simulink library "motion"  (Simulink 4.00)
undefined symbols (not defined in the file or in its folder): A6, Ac, Acd, ad, Aff, Aff0, Aff6, Ap, As, B6, Bc, Bcd, Bff, Bff0, Bff6, Bp, Bs, C6, Cc, Ccd, Cff, Cff0, Cff6, Cp, Cs, D6, Dc, dd, Ddd, Dff, Dff0, Dff6, Dp, Ds, jd, Ts, Tsettle
libraries: motion x5
(part 4 of 4)

== system motion/Real Time/Plan Trajectory (with displays)/Round up7 ==
  In1 : Inport  Port=1
  Product : Product  Inputs=*/  Multiplication=Element-wise(.*)  SaturateOnIntegerOverflow=on
  Product1 : Product  Inputs=**  Multiplication=Element-wise(.*)  SaturateOnIntegerOverflow=on
  Round up : Rounding  Operator=ceil
  Out1 : Outport  Port=1
  wires:
  [Ts] -> Product1/2, Product/2
  Product/1 -> Round up/1
  Round up/1 -> Product1/1
  In1/1 -> Product/1
  Product1/1 -> Out1/1

== system motion/Real Time/Plan Trajectory (with displays)/Round up8 ==
  In1 : Inport  Port=1
  Product : Product  Inputs=*/  Multiplication=Element-wise(.*)  SaturateOnIntegerOverflow=on
  Product1 : Product  Inputs=**  Multiplication=Element-wise(.*)  SaturateOnIntegerOverflow=on
  Round up : Rounding  Operator=ceil
  Out1 : Outport  Port=1
  wires:
  Product1/1 -> Out1/1
  In1/1 -> Product/1
  Round up/1 -> Product1/1
  Product/1 -> Round up/1
  [Ts] -> Product/2, Product1/2

== system motion/Real Time/Plan Trajectory (with displays)/Round up9 ==
  In1 : Inport  Port=1
  Product : Product  Inputs=*/  Multiplication=Element-wise(.*)  SaturateOnIntegerOverflow=on
  Product1 : Product  Inputs=**  Multiplication=Element-wise(.*)  SaturateOnIntegerOverflow=on
  Round up : Rounding  Operator=ceil
  Out1 : Outport  Port=1
  wires:
  [Ts] -> Product1/2, Product/2
  Product/1 -> Round up/1
  Round up/1 -> Product1/1
  In1/1 -> Product/1
  Product1/1 -> Out1/1

== system motion/Real Time/Plan Trajectory (with displays)/ta amax ==
  u : Inport  Port=1
  dd : Inport  Port=2
  Mux1 : Mux  Inputs=3
  Mux17 : Mux  Inputs=3
  c1 : Fcn  Expr=u(1)*(u(1)+u(2))
  c2 : Fcn  Expr=3*u(1)*( 2*u(1)^2 + u(2)*(3*u(1) + u(2)) )
  c3 : Fcn  Expr=2*u(1)*( u(1)*( 4*u(1)^2 + u(2)*(8*u(1) + 5*u(2)) ) + u(2)^3 )
  ta calc : Fcn  Expr=(-u(10) + sqrt(u(10)^2-4*u(9)*(u(11)-u(1)/u(8))))/(2*u(9))
  ta : Outport  Port=1
  c : Outport  Port=2
  wires:
  [dd] -> Mux1/2
  Mux17/1 -> c/1, [c]
  c1/1 -> Mux17/1
  c3/1 -> Mux17/3
  c2/1 -> Mux17/2
  ta calc/1 -> ta/1
  [c] -> Mux1/3
  [u] -> Mux1/1
  Mux1/1 -> ta calc/1
  [dd] -> c3/1, c2/1, c1/1
  dd/1 -> [dd]
  u/1 -> [u]

== system motion/Real Time/Plan Trajectory (with displays)/tj jmax ==
  u : Inport  Port=1
  dd : Inport  Port=2
  D : Fcn  Expr=sqrt(u(1)^3+u(2)^2)
  Demux : Demux  Outputs=5  BusSelectionMode=off
  Demux1 : Demux  Outputs=2  BusSelectionMode=off
  Mux1 : Mux  Inputs=2
  Mux12 : Mux  Inputs=2
  Mux2 : Mux  Inputs=2
  Mux3 : Mux  Inputs=3
  P : Fcn  Expr=-1/9*u(1)^2
  Q : Fcn  Expr=-1/27*u(1)^3-u(3)/(4*u(2)*u(1))
  R : Fcn  Expr=(-u(1)+u(2))^(1/3)
  Terminator{,1..4} (5 alike) : Terminator
  tj calc : Fcn  Expr=u(2) - u(1)/u(2) - 5/3*u(3)
  tj : Outport  Port=1
  wires:
  [td] -> Mux3/3
  tj calc/1 -> tj/1
  [R] -> Mux3/2
  [P] -> Mux3/1
  Mux3/1 -> tj calc/1
  R/1 -> [R]
  [D] -> Mux2/2
  [Q] -> Mux2/1
  Mux2/1 -> R/1
  D/1 -> [D]
  [Q] -> Mux1/2
  [P] -> Mux1/1
  Mux1/1 -> D/1
  Q/1 -> [Q]
  P/1 -> [P]
  [p] -> Mux12/2
  Mux12/1 -> Q/1
  [dd] -> Mux12/1, P/1
  Demux1/1 -> [td]
  Demux1/2 -> Terminator4/1  "dd"
  dd/1 -> [dd], Demux1/1
  Demux/5 -> Terminator3/1  "d"
  Demux/4 -> Terminator/1  "j"
  Demux/3 -> Terminator1/1  "a"
  Demux/2 -> Terminator2/1  "v"
  Demux/1 -> [p]
  u/1 -> Demux/1

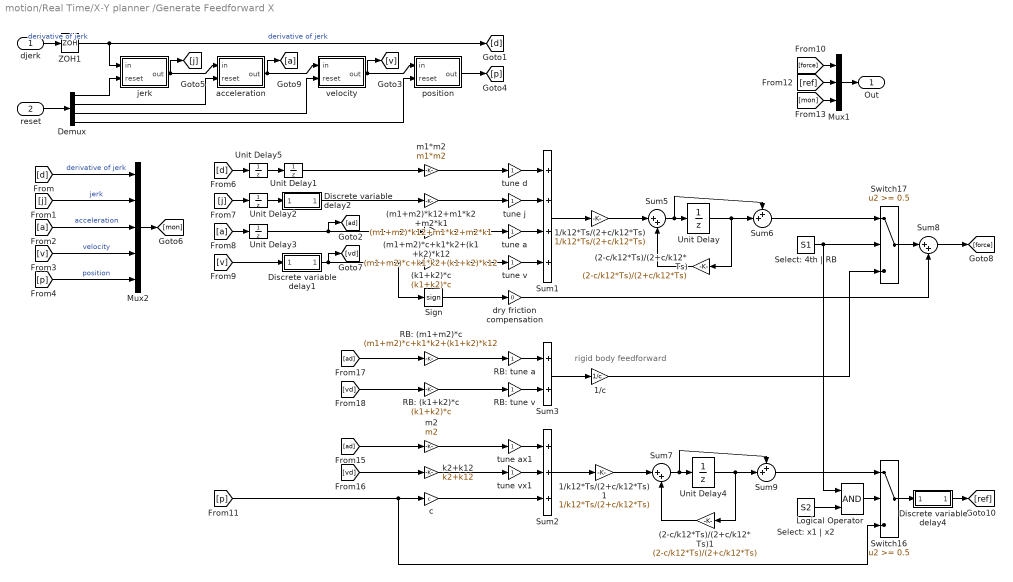
== system motion/Real Time/X-Y planner /Generate Feedforward X ==
  note: rigid body feedforward
  djerk : Inport  Port=1
  reset : Inport  Port=2
  (2-c/k12*Ts)/(2+c/k12*Ts) : Gain  Orientation=left  Gain=(2-c/k12*Ts)/(2+c/k12*Ts)  Multiplication=Element-wise(K.*u)  SaturateOnIntegerOverflow=on
  (2-c/k12*Ts)/(2+c/k12*Ts)1 : Gain  Orientation=left  Gain=(2-c/k12*Ts)/(2+c/k12*Ts)  Multiplication=Element-wise(K.*u)  SaturateOnIntegerOverflow=on
  (k1+k2)*c : Gain  Gain=(k1+k2)*c  Multiplication=Element-wise(K.*u)  SaturateOnIntegerOverflow=on
  (m1+m2)*c+k1*k2+(k1+k2)*k12 : Gain  Gain=(m1+m2)*c+k1*k2+(k1+k2)*k12  Multiplication=Element-wise(K.*u)  SaturateOnIntegerOverflow=on
  (m1+m2)*k12+m1*k2+m2*k1 : Gain  Gain=(m1+m2)*k12+m1*k2+m2*k1  Multiplication=Element-wise(K.*u)  SaturateOnIntegerOverflow=on
  1/c : Gain  Gain=1/c  Multiplication=Element-wise(K.*u)  SaturateOnIntegerOverflow=on
  1/k12*Ts/(2+c/k12*Ts) : Gain  Gain=1/k12*Ts/(2+c/k12*Ts)  Multiplication=Element-wise(K.*u)  SaturateOnIntegerOverflow=on
  1/k12*Ts/(2+c/k12*Ts)1 : Gain  Gain=1/k12*Ts/(2+c/k12*Ts)  Multiplication=Element-wise(K.*u)  SaturateOnIntegerOverflow=on
  Demux : Demux  Outputs=4  BusSelectionMode=off
  Discrete variable delay1 : Subsystem  mask{Ts=Ts, alpha=.5}
      mask prompts: Ts "Sample time"; alpha "Delay factor (between 0 and 1)"
      settings: RTWFcnNameOpts=Auto  RTWFileNameOpts=Auto
      mask Display: disp(sprintf('%3.1f*Ts',alpha))
  Discrete variable delay2 : Subsystem  mask{Ts=Ts, alpha=.5}
      mask prompts: Ts "Sample time"; alpha "Delay factor (between 0 and 1)"
      settings: RTWFcnNameOpts=Auto  RTWFileNameOpts=Auto
      mask Display: disp(sprintf('%3.1f*Ts',alpha))
  Discrete variable delay4 : Subsystem  mask{Ts=Ts, alpha=.5}
      mask prompts: Ts "Sample time"; alpha "Delay factor (between 0 and 1)"
      settings: RTWFcnNameOpts=Auto  RTWFileNameOpts=Auto
      mask Display: disp(sprintf('%3.1f*Ts',alpha))
  Logical Operator : Logic  Operator=AND  Inputs=2
  Mux1 : Mux  Inputs=3
  Mux2 : Mux  Inputs=5
  RB: (k1+k2)*c : Gain  Gain=(k1+k2)*c  Multiplication=Element-wise(K.*u)  SaturateOnIntegerOverflow=on
  RB: (m1+m2)*c : Gain  Gain=(m1+m2)*c+k1*k2+(k1+k2)*k12  Multiplication=Element-wise(K.*u)  SaturateOnIntegerOverflow=on
  RB: tune a : Gain  Gain=1  Multiplication=Element-wise(K.*u)  SaturateOnIntegerOverflow=on
  RB: tune v : Gain  Gain=1  Multiplication=Element-wise(K.*u)  SaturateOnIntegerOverflow=on
  Select: 4th | RB : Constant  Value=S1
  Select: x1 | x2 : Constant  Value=S2
  Sign : Signum
  Sum1 : Sum  Inputs=++++  SaturateOnIntegerOverflow=on
  Sum2 : Sum  Inputs=+++  SaturateOnIntegerOverflow=on
  Sum3 : Sum  Inputs=++  SaturateOnIntegerOverflow=on
  Sum5 : Sum  Inputs=|++  SaturateOnIntegerOverflow=on
  Sum6 : Sum  Inputs=++|  SaturateOnIntegerOverflow=on
  Sum7 : Sum  Inputs=|++  SaturateOnIntegerOverflow=on
  Sum8 : Sum  Inputs=|++  SaturateOnIntegerOverflow=on
  Sum9 : Sum  Inputs=++|  SaturateOnIntegerOverflow=on
  Switch16 : Switch  Threshold=0.5
  Switch17 : Switch  Threshold=0.5
  Unit Delay{,1..5} (6 alike) : UnitDelay  X0=0  SampleTime=Ts
  ZOH1 : ZeroOrderHold  SampleTime=Ts
  acceleration : Subsystem
      settings: RTWFcnNameOpts=Auto  RTWFileNameOpts=Auto
  c : Gain  Gain=c  Multiplication=Element-wise(K.*u)  SaturateOnIntegerOverflow=on
  dry friction compensation : Gain  Gain=0  Multiplication=Element-wise(K.*u)  SaturateOnIntegerOverflow=on
  jerk : Subsystem
      settings: RTWFcnNameOpts=Auto  RTWFileNameOpts=Auto
  k2+k12 : Gain  Gain=k2+k12  Multiplication=Element-wise(K.*u)  SaturateOnIntegerOverflow=on
  m1*m2 : Gain  Gain=m1*m2  Multiplication=Element-wise(K.*u)  SaturateOnIntegerOverflow=on
  m2 : Gain  Gain=m2  Multiplication=Element-wise(K.*u)  SaturateOnIntegerOverflow=on
  position : Subsystem
      settings: RTWFcnNameOpts=Auto  RTWFileNameOpts=Auto
  tune a : Gain  Gain=1  Multiplication=Element-wise(K.*u)  SaturateOnIntegerOverflow=on
  tune ax1 : Gain  Gain=1  Multiplication=Element-wise(K.*u)  SaturateOnIntegerOverflow=on
  tune d : Gain  Gain=1  Multiplication=Element-wise(K.*u)  SaturateOnIntegerOverflow=on
  tune j : Gain  Gain=1  Multiplication=Element-wise(K.*u)  SaturateOnIntegerOverflow=on
  tune v : Gain  Gain=1  Multiplication=Element-wise(K.*u)  SaturateOnIntegerOverflow=on
  tune vx1 : Gain  Gain=1  Multiplication=Element-wise(K.*u)  SaturateOnIntegerOverflow=on
  velocity : Subsystem
      settings: RTWFcnNameOpts=Auto  RTWFileNameOpts=Auto
  Out : Outport  Port=1
  wires:
  c/1 -> Sum2/3
  Select: 4th | RB/1 -> Logical Operator/1, Switch17/2
  Sum9/1 -> Switch16/1
  1/c/1 -> Switch17/3
  dry friction compensation/1 -> Sum8/2
  Logical Operator/1 -> Switch16/2
  Select: x1 | x2/1 -> Logical Operator/2
  Discrete variable delay4/1(Out1) -> [ref]
  Switch16/1 -> Discrete variable delay4/1(In1)
  Sum8/1 -> [force]
  Switch17/1 -> Sum8/1
  Sum6/1 -> Switch17/1
  Unit Delay4/1 -> Sum9/2, (2-c/k12*Ts)/(2+c/k12*Ts)1/1
  Sum7/1 -> Sum9/1, Unit Delay4/1
  1/k12*Ts/(2+c/k12*Ts)1/1 -> Sum7/1
  Sum2/1 -> 1/k12*Ts/(2+c/k12*Ts)1/1
  (2-c/k12*Ts)/(2+c/k12*Ts)1/1 -> Sum7/2
  [vd] -> k2+k12/1
  [ad] -> m2/1
  [p] -> c/1, Switch16/3
  m2/1 -> tune ax1/1
  tune ax1/1 -> Sum2/1
  k2+k12/1 -> tune vx1/1
  tune vx1/1 -> Sum2/2
  [ad] -> RB: (m1+m2)*c/1
  [vd] -> RB: (k1+k2)*c/1
  RB: (m1+m2)*c/1 -> RB: tune a/1
  RB: tune a/1 -> Sum3/1
  RB: (k1+k2)*c/1 -> RB: tune v/1
  RB: tune v/1 -> Sum3/2
  Sum3/1 -> 1/c/1
  [force] -> Mux1/1
  [ref] -> Mux1/2
  [mon] -> Mux1/3
  Mux1/1 -> Out/1
  Unit Delay3/1 -> [ad], (m1+m2)*c+k1*k2+(k1+k2)*k12/1
  Discrete variable delay2/1(Out1) -> (m1+m2)*k12+m1*k2+m2*k1/1
  Unit Delay1/1 -> m1*m2/1
  m1*m2/1 -> tune d/1
  tune d/1 -> Sum1/1
  (m1+m2)*k12+m1*k2+m2*k1/1 -> tune j/1
  tune j/1 -> Sum1/2
  (m1+m2)*c+k1*k2+(k1+k2)*k12/1 -> tune a/1
  tune a/1 -> Sum1/3
  (k1+k2)*c/1 -> tune v/1
  tune v/1 -> Sum1/4
  Unit Delay/1 -> Sum6/2, (2-c/k12*Ts)/(2+c/k12*Ts)/1
  Sum5/1 -> Sum6/1, Unit Delay/1
  1/k12*Ts/(2+c/k12*Ts)/1 -> Sum5/1
  Sum1/1 -> 1/k12*Ts/(2+c/k12*Ts)/1
  (2-c/k12*Ts)/(2+c/k12*Ts)/1 -> Sum5/2
  Sign/1 -> dry friction compensation/1
  djerk/1 -> ZOH1/1  "derivative of jerk"
  Unit Delay2/1 -> Discrete variable delay2/1(In1)
  Unit Delay5/1 -> Unit Delay1/1
  [v] -> Discrete variable delay1/1(In1)
  [a] -> Unit Delay3/1
  [j] -> Unit Delay2/1
  [d] -> Unit Delay5/1
  [v] -> Mux2/4  "velocity"
  [a] -> Mux2/3  "acceleration"
  [j] -> Mux2/2  "jerk"
  [d] -> Mux2/1  "derivative of jerk"
  [p] -> Mux2/5  "position"
  Mux2/1 -> [mon]
  reset/1 -> Demux/1
  ZOH1/1 -> jerk/1(in), [d]  "derivative of jerk"
  acceleration/1(out) -> [a], velocity/1(in)
  jerk/1(out) -> [j], acceleration/1(in)
  Demux/1 -> jerk/2(reset)
  Demux/2 -> acceleration/2(reset)
  Demux/3 -> velocity/2(reset)
  velocity/1(out) -> [v], position/1(in)
  Demux/4 -> position/2(reset)
  Discrete variable delay1/1(Out1) -> [vd], (k1+k2)*c/1, Sign/1
  position/1(out) -> [p]

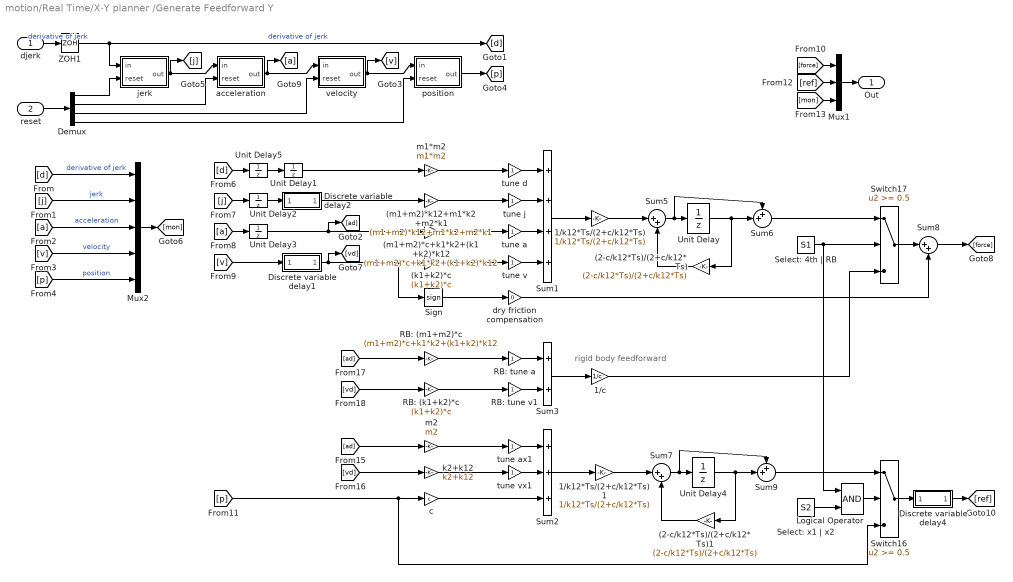
== system motion/Real Time/X-Y planner /Generate Feedforward Y ==
  note: rigid body feedforward
  djerk : Inport  Port=1
  reset : Inport  Port=2
  (2-c/k12*Ts)/(2+c/k12*Ts) : Gain  Orientation=left  Gain=(2-c/k12*Ts)/(2+c/k12*Ts)  Multiplication=Element-wise(K.*u)  SaturateOnIntegerOverflow=on
  (2-c/k12*Ts)/(2+c/k12*Ts)1 : Gain  Orientation=left  Gain=(2-c/k12*Ts)/(2+c/k12*Ts)  Multiplication=Element-wise(K.*u)  SaturateOnIntegerOverflow=on
  (k1+k2)*c : Gain  Gain=(k1+k2)*c  Multiplication=Element-wise(K.*u)  SaturateOnIntegerOverflow=on
  (m1+m2)*c+k1*k2+(k1+k2)*k12 : Gain  Gain=(m1+m2)*c+k1*k2+(k1+k2)*k12  Multiplication=Element-wise(K.*u)  SaturateOnIntegerOverflow=on
  (m1+m2)*k12+m1*k2+m2*k1 : Gain  Gain=(m1+m2)*k12+m1*k2+m2*k1  Multiplication=Element-wise(K.*u)  SaturateOnIntegerOverflow=on
  1/c : Gain  Gain=1/c  Multiplication=Element-wise(K.*u)  SaturateOnIntegerOverflow=on
  1/k12*Ts/(2+c/k12*Ts) : Gain  Gain=1/k12*Ts/(2+c/k12*Ts)  Multiplication=Element-wise(K.*u)  SaturateOnIntegerOverflow=on
  1/k12*Ts/(2+c/k12*Ts)1 : Gain  Gain=1/k12*Ts/(2+c/k12*Ts)  Multiplication=Element-wise(K.*u)  SaturateOnIntegerOverflow=on
  Demux : Demux  Outputs=4  BusSelectionMode=off
  Discrete variable delay1 : Subsystem  mask{Ts=Ts, alpha=.5}
      mask prompts: Ts "Sample time"; alpha "Delay factor (between 0 and 1)"
      settings: RTWFcnNameOpts=Auto  RTWFileNameOpts=Auto
      mask Display: disp(sprintf('%3.1f*Ts',alpha))
  Discrete variable delay2 : Subsystem  mask{Ts=Ts, alpha=.5}
      mask prompts: Ts "Sample time"; alpha "Delay factor (between 0 and 1)"
      settings: RTWFcnNameOpts=Auto  RTWFileNameOpts=Auto
      mask Display: disp(sprintf('%3.1f*Ts',alpha))
  Discrete variable delay4 : Subsystem  mask{Ts=Ts, alpha=.5}
      mask prompts: Ts "Sample time"; alpha "Delay factor (between 0 and 1)"
      settings: RTWFcnNameOpts=Auto  RTWFileNameOpts=Auto
      mask Display: disp(sprintf('%3.1f*Ts',alpha))
  Logical Operator : Logic  Operator=AND  Inputs=2
  Mux1 : Mux  Inputs=3
  Mux2 : Mux  Inputs=5
  RB: (k1+k2)*c : Gain  Gain=(k1+k2)*c  Multiplication=Element-wise(K.*u)  SaturateOnIntegerOverflow=on
  RB: (m1+m2)*c : Gain  Gain=(m1+m2)*c+k1*k2+(k1+k2)*k12  Multiplication=Element-wise(K.*u)  SaturateOnIntegerOverflow=on
  RB: tune a : Gain  Gain=1  Multiplication=Element-wise(K.*u)  SaturateOnIntegerOverflow=on
  RB: tune v1 : Gain  Gain=1  Multiplication=Element-wise(K.*u)  SaturateOnIntegerOverflow=on
  Select: 4th | RB : Constant  Value=S1
  Select: x1 | x2 : Constant  Value=S2
  Sign : Signum
  Sum1 : Sum  Inputs=++++  SaturateOnIntegerOverflow=on
  Sum2 : Sum  Inputs=+++  SaturateOnIntegerOverflow=on
  Sum3 : Sum  Inputs=++  SaturateOnIntegerOverflow=on
  Sum5 : Sum  Inputs=|++  SaturateOnIntegerOverflow=on
  Sum6 : Sum  Inputs=++|  SaturateOnIntegerOverflow=on
  Sum7 : Sum  Inputs=|++  SaturateOnIntegerOverflow=on
  Sum8 : Sum  Inputs=|++  SaturateOnIntegerOverflow=on
  Sum9 : Sum  Inputs=++|  SaturateOnIntegerOverflow=on
  Switch16 : Switch  Threshold=0.5
  Switch17 : Switch  Threshold=0.5
  Unit Delay{,1..5} (6 alike) : UnitDelay  X0=0  SampleTime=Ts
  ZOH1 : ZeroOrderHold  SampleTime=Ts
  acceleration : Subsystem
      settings: RTWFcnNameOpts=Auto  RTWFileNameOpts=Auto
  c : Gain  Gain=c  Multiplication=Element-wise(K.*u)  SaturateOnIntegerOverflow=on
  dry friction compensation : Gain  Gain=0  Multiplication=Element-wise(K.*u)  SaturateOnIntegerOverflow=on
  jerk : Subsystem
      settings: RTWFcnNameOpts=Auto  RTWFileNameOpts=Auto
  k2+k12 : Gain  Gain=k2+k12  Multiplication=Element-wise(K.*u)  SaturateOnIntegerOverflow=on
  m1*m2 : Gain  Gain=m1*m2  Multiplication=Element-wise(K.*u)  SaturateOnIntegerOverflow=on
  m2 : Gain  Gain=m2  Multiplication=Element-wise(K.*u)  SaturateOnIntegerOverflow=on
  position : Subsystem
      settings: RTWFcnNameOpts=Auto  RTWFileNameOpts=Auto
  tune a : Gain  Gain=1  Multiplication=Element-wise(K.*u)  SaturateOnIntegerOverflow=on
  tune ax1 : Gain  Gain=1  Multiplication=Element-wise(K.*u)  SaturateOnIntegerOverflow=on
  tune d : Gain  Gain=1  Multiplication=Element-wise(K.*u)  SaturateOnIntegerOverflow=on
  tune j : Gain  Gain=1  Multiplication=Element-wise(K.*u)  SaturateOnIntegerOverflow=on
  tune v : Gain  Gain=1  Multiplication=Element-wise(K.*u)  SaturateOnIntegerOverflow=on
  tune vx1 : Gain  Gain=1  Multiplication=Element-wise(K.*u)  SaturateOnIntegerOverflow=on
  velocity : Subsystem
      settings: RTWFcnNameOpts=Auto  RTWFileNameOpts=Auto
  Out : Outport  Port=1
  wires:
  position/1(out) -> [p]
  Discrete variable delay1/1(Out1) -> Sign/1, (k1+k2)*c/1, [vd]
  Demux/4 -> position/2(reset)
  velocity/1(out) -> position/1(in), [v]
  Demux/3 -> velocity/2(reset)
  Demux/2 -> acceleration/2(reset)
  Demux/1 -> jerk/2(reset)
  jerk/1(out) -> acceleration/1(in), [j]
  acceleration/1(out) -> velocity/1(in), [a]
  ZOH1/1 -> [d], jerk/1(in)  "derivative of jerk"
  reset/1 -> Demux/1
  Mux2/1 -> [mon]
  [p] -> Mux2/5  "position"
  [d] -> Mux2/1  "derivative of jerk"
  [j] -> Mux2/2  "jerk"
  [a] -> Mux2/3  "acceleration"
  [v] -> Mux2/4  "velocity"
  [d] -> Unit Delay5/1
  [j] -> Unit Delay2/1
  [a] -> Unit Delay3/1
  [v] -> Discrete variable delay1/1(In1)
  Unit Delay5/1 -> Unit Delay1/1
  Unit Delay2/1 -> Discrete variable delay2/1(In1)
  djerk/1 -> ZOH1/1  "derivative of jerk"
  Sign/1 -> dry friction compensation/1
  (2-c/k12*Ts)/(2+c/k12*Ts)/1 -> Sum5/2
  Sum1/1 -> 1/k12*Ts/(2+c/k12*Ts)/1
  1/k12*Ts/(2+c/k12*Ts)/1 -> Sum5/1
  Sum5/1 -> Unit Delay/1, Sum6/1
  Unit Delay/1 -> (2-c/k12*Ts)/(2+c/k12*Ts)/1, Sum6/2
  tune v/1 -> Sum1/4
  (k1+k2)*c/1 -> tune v/1
  tune a/1 -> Sum1/3
  (m1+m2)*c+k1*k2+(k1+k2)*k12/1 -> tune a/1
  tune j/1 -> Sum1/2
  (m1+m2)*k12+m1*k2+m2*k1/1 -> tune j/1
  tune d/1 -> Sum1/1
  m1*m2/1 -> tune d/1
  Unit Delay1/1 -> m1*m2/1
  Discrete variable delay2/1(Out1) -> (m1+m2)*k12+m1*k2+m2*k1/1
  Unit Delay3/1 -> (m1+m2)*c+k1*k2+(k1+k2)*k12/1, [ad]
  Mux1/1 -> Out/1
  [mon] -> Mux1/3
  [ref] -> Mux1/2
  [force] -> Mux1/1
  Sum3/1 -> 1/c/1
  RB: tune v1/1 -> Sum3/2
  RB: (k1+k2)*c/1 -> RB: tune v1/1
  RB: tune a/1 -> Sum3/1
  RB: (m1+m2)*c/1 -> RB: tune a/1
  [vd] -> RB: (k1+k2)*c/1
  [ad] -> RB: (m1+m2)*c/1
  tune vx1/1 -> Sum2/2
  k2+k12/1 -> tune vx1/1
  tune ax1/1 -> Sum2/1
  m2/1 -> tune ax1/1
  [p] -> Switch16/3, c/1
  [ad] -> m2/1
  [vd] -> k2+k12/1
  (2-c/k12*Ts)/(2+c/k12*Ts)1/1 -> Sum7/2
  Sum2/1 -> 1/k12*Ts/(2+c/k12*Ts)1/1
  1/k12*Ts/(2+c/k12*Ts)1/1 -> Sum7/1
  Sum7/1 -> Unit Delay4/1, Sum9/1
  Unit Delay4/1 -> (2-c/k12*Ts)/(2+c/k12*Ts)1/1, Sum9/2
  Sum6/1 -> Switch17/1
  Switch17/1 -> Sum8/1
  Sum8/1 -> [force]
  Switch16/1 -> Discrete variable delay4/1(In1)
  Discrete variable delay4/1(Out1) -> [ref]
  Select: x1 | x2/1 -> Logical Operator/2
  Logical Operator/1 -> Switch16/2
  dry friction compensation/1 -> Sum8/2
  1/c/1 -> Switch17/3
  Sum9/1 -> Switch16/1
  Select: 4th | RB/1 -> Switch17/2, Logical Operator/1
  c/1 -> Sum2/3

== system motion/Real Time/X-Y planner /Waypoints ==
  start position : Inport  Port=1
  Trigger : TriggerPort  TriggerType=rising  OutputDataType=auto
  0 : Memory  X0=0  InheritSampleTime=on
  Constant1 : Constant  Value=pmin
  Constant2 : Constant  Value=1
  Constant3 : Constant  Value=0
  Constant4 : Constant  Value=0
  Memory : Memory  X0=0  InheritSampleTime=on
  Mux1 : Mux  Inputs=2
  Relational Operator : RelationalOperator  Operator=>
  Sum3 : Sum  Inputs=|+-  SaturateOnIntegerOverflow=on
  Switch{1..4} (4 alike) : Switch  Threshold=0.5
  distance : Fcn  Expr=sqrt( u(1)^2 + u(2)^2 )
  factor X : Fcn  Expr=u(2)/u(1)
  factor Y : Fcn  Expr=u(3)/u(1)
  positions : FromWorkspace  VariableName=X  SampleTime=-1  Interpolate=off  OutputAfterFinalValue=CyclicRepetition
  p : Outport  Port=1
  X : Outport  Port=2
  Y : Outport  Port=3
  pos : Outport  Port=4
  wires:
  Constant1/1 -> Switch4/1, Relational Operator/1
  Switch3/1 -> Y/1
  Switch2/1 -> X/1
  Switch4/1 -> p/1
  Relational Operator/1 -> Switch4/2, Switch3/2, Switch2/2
  Constant4/1 -> Switch3/1
  Constant3/1 -> Switch2/1
  factor Y/1 -> Switch3/3
  factor X/1 -> Switch2/3
  Switch1/1 -> Sum3/2
  Sum3/1 -> Mux1/2, distance/1
  Memory/1 -> Switch1/1
  start position/1 -> Switch1/3
  positions/1 -> pos/1, Memory/1, Sum3/1
  Mux1/1 -> factor Y/1, factor X/1
  distance/1 -> Switch4/3, Relational Operator/2, Mux1/1
  Constant2/1 -> 0/1
  0/1 -> Switch1/2

== system motion/Real Time/X-Y planner /single move  ==
  trigger : Inport  Port=1
  start : Inport  Port=2
  0 : Constant  Value=0
  0/1 : Saturate  UpperLimit=1  LowerLimit=0  LinearizeAsGain=on
  Logical Operator3 : Logic  Operator=OR  Inputs=2
  Memory1 : Memory  X0=0  InheritSampleTime=on
  Memory2 : Memory  X0=0  InheritSampleTime=on
  Sum : Sum  Inputs=|+-  SaturateOnIntegerOverflow=on
  Switch1 : Switch  Threshold=.5
  enable : Outport  Port=1
  wires:
  0/1 -> Switch1/1
  Switch1/1 -> Memory2/1
  start/1 -> Switch1/2
  0/1/1 -> Logical Operator3/1
  Logical Operator3/1 -> Switch1/3
  Memory2/1 -> Logical Operator3/2, enable/1
  trigger/1 -> Memory1/1, Sum/1
  Memory1/1 -> Sum/2
  Sum/1 -> 0/1/1

== system motion/Real Time/X-Y planner /Generate Feedforward X/Discrete variable delay1 ==
  In1 : Inport  Port=1
  1-alpha : Gain  Gain=1-alpha  Multiplication=Element-wise(K.*u)  SaturateOnIntegerOverflow=on
  Sum1 : Sum  Inputs=++|  SaturateOnIntegerOverflow=on
  Sum2 : Sum  Inputs=+-|  SaturateOnIntegerOverflow=on
  Unit Delay : UnitDelay  X0=0  SampleTime=Ts
  Out1 : Outport  Port=1
  wires:
  In1/1 -> Sum2/1, Unit Delay/1
  Unit Delay/1 -> Sum1/2, Sum2/2
  Sum1/1 -> Out1/1
  1-alpha/1 -> Sum1/1
  Sum2/1 -> 1-alpha/1

== system motion/Real Time/X-Y planner /Generate Feedforward X/Discrete variable delay2 ==
  In1 : Inport  Port=1
  1-alpha : Gain  Gain=1-alpha  Multiplication=Element-wise(K.*u)  SaturateOnIntegerOverflow=on
  Sum1 : Sum  Inputs=++|  SaturateOnIntegerOverflow=on
  Sum2 : Sum  Inputs=+-|  SaturateOnIntegerOverflow=on
  Unit Delay : UnitDelay  X0=0  SampleTime=Ts
  Out1 : Outport  Port=1
  wires:
  Sum2/1 -> 1-alpha/1
  1-alpha/1 -> Sum1/1
  Sum1/1 -> Out1/1
  Unit Delay/1 -> Sum2/2, Sum1/2
  In1/1 -> Unit Delay/1, Sum2/1

== system motion/Real Time/X-Y planner /Generate Feedforward X/Discrete variable delay4 ==
  In1 : Inport  Port=1
  1-alpha : Gain  Gain=1-alpha  Multiplication=Element-wise(K.*u)  SaturateOnIntegerOverflow=on
  Sum1 : Sum  Inputs=++|  SaturateOnIntegerOverflow=on
  Sum2 : Sum  Inputs=+-|  SaturateOnIntegerOverflow=on
  Unit Delay : UnitDelay  X0=0  SampleTime=Ts
  Out1 : Outport  Port=1
  wires:
  In1/1 -> Sum2/1, Unit Delay/1
  Unit Delay/1 -> Sum1/2, Sum2/2
  Sum1/1 -> Out1/1
  1-alpha/1 -> Sum1/1
  Sum2/1 -> 1-alpha/1

== system motion/Real Time/X-Y planner /Generate Feedforward X/acceleration ==
  in : Inport  Port=1
  reset : Inport  Port=2
  Constant : Constant  Value=0
  Constant1 : Constant  Value=0
  Gain4 : Gain  Gain=Ts/2  Multiplication=Element-wise(K.*u)  SaturateOnIntegerOverflow=on
  Sum : Sum  Inputs=|++  SaturateOnIntegerOverflow=on
  Sum1 : Sum  Inputs=|-+  SaturateOnIntegerOverflow=on
  Sum6 : Sum  Inputs=+-  SaturateOnIntegerOverflow=on
  Switch : Switch  Threshold=.5
  Switch1 : Switch  Threshold=.5
  Unit Delay4 : UnitDelay  X0=0  SampleTime=Ts
  Unit Delay5 : UnitDelay  X0=0  SampleTime=Ts
  out : Outport  Port=1
  wires:
  Unit Delay4/1 -> Sum/2, Sum6/1
  Switch1/1 -> Unit Delay5/1
  Switch/1 -> Unit Delay4/1
  Unit Delay5/1 -> Sum6/2, Sum1/2
  Sum6/1 -> out/1
  in/1 -> Gain4/1
  Gain4/1 -> Sum1/1, Sum/1
  Sum1/1 -> Switch1/3
  Constant1/1 -> Switch1/1
  reset/1 -> Switch1/2, Switch/2
  Sum/1 -> Switch/3
  Constant/1 -> Switch/1

== system motion/Real Time/X-Y planner /Generate Feedforward X/jerk ==
  in : Inport  Port=1
  reset : Inport  Port=2
  Constant : Constant  Value=0
  Constant1 : Constant  Value=0
  Gain4 : Gain  Gain=Ts/2  Multiplication=Element-wise(K.*u)  SaturateOnIntegerOverflow=on
  Sum : Sum  Inputs=|++  SaturateOnIntegerOverflow=on
  Sum1 : Sum  Inputs=|-+  SaturateOnIntegerOverflow=on
  Sum6 : Sum  Inputs=+-  SaturateOnIntegerOverflow=on
  Switch : Switch  Threshold=.5
  Switch1 : Switch  Threshold=.5
  Unit Delay4 : UnitDelay  X0=0  SampleTime=Ts
  Unit Delay5 : UnitDelay  X0=0  SampleTime=Ts
  out : Outport  Port=1
  wires:
  Constant/1 -> Switch/1
  Sum/1 -> Switch/3
  reset/1 -> Switch/2, Switch1/2
  Constant1/1 -> Switch1/1
  Sum1/1 -> Switch1/3
  Gain4/1 -> Sum/1, Sum1/1
  in/1 -> Gain4/1
  Sum6/1 -> out/1
  Unit Delay5/1 -> Sum1/2, Sum6/2
  Switch/1 -> Unit Delay4/1
  Switch1/1 -> Unit Delay5/1
  Unit Delay4/1 -> Sum6/1, Sum/2

== system motion/Real Time/X-Y planner /Generate Feedforward X/position ==
  in : Inport  Port=1
  reset : Inport  Port=2
  Constant : Constant  Value=0
  Constant1 : Constant  Value=0
  Gain4 : Gain  Gain=Ts/2  Multiplication=Element-wise(K.*u)  SaturateOnIntegerOverflow=on
  Sum : Sum  Inputs=|++  SaturateOnIntegerOverflow=on
  Sum1 : Sum  Inputs=|-+  SaturateOnIntegerOverflow=on
  Sum6 : Sum  Inputs=+-  SaturateOnIntegerOverflow=on
  Switch : Switch  Threshold=.5
  Switch1 : Switch  Threshold=.5
  Unit Delay4 : UnitDelay  X0=0  SampleTime=Ts
  Unit Delay5 : UnitDelay  X0=0  SampleTime=Ts
  out : Outport  Port=1
  wires:
  Unit Delay4/1 -> Sum/2, Sum6/1
  Switch1/1 -> Unit Delay5/1
  Switch/1 -> Unit Delay4/1
  Unit Delay5/1 -> Sum6/2, Sum1/2
  Sum6/1 -> out/1
  in/1 -> Gain4/1
  Gain4/1 -> Sum1/1, Sum/1
  Sum1/1 -> Switch1/3
  Constant1/1 -> Switch1/1
  reset/1 -> Switch1/2, Switch/2
  Sum/1 -> Switch/3
  Constant/1 -> Switch/1

== system motion/Real Time/X-Y planner /Generate Feedforward X/velocity ==
  in : Inport  Port=1
  reset : Inport  Port=2
  Constant : Constant  Value=0
  Constant1 : Constant  Value=0
  Gain4 : Gain  Gain=Ts/2  Multiplication=Element-wise(K.*u)  SaturateOnIntegerOverflow=on
  Sum : Sum  Inputs=|++  SaturateOnIntegerOverflow=on
  Sum1 : Sum  Inputs=|-+  SaturateOnIntegerOverflow=on
  Sum6 : Sum  Inputs=+-  SaturateOnIntegerOverflow=on
  Switch : Switch  Threshold=.5
  Switch1 : Switch  Threshold=.5
  Unit Delay4 : UnitDelay  X0=0  SampleTime=Ts
  Unit Delay5 : UnitDelay  X0=0  SampleTime=Ts
  out : Outport  Port=1
  wires:
  Constant/1 -> Switch/1
  Sum/1 -> Switch/3
  reset/1 -> Switch/2, Switch1/2
  Constant1/1 -> Switch1/1
  Sum1/1 -> Switch1/3
  Gain4/1 -> Sum/1, Sum1/1
  in/1 -> Gain4/1
  Sum6/1 -> out/1
  Unit Delay5/1 -> Sum1/2, Sum6/2
  Switch/1 -> Unit Delay4/1
  Switch1/1 -> Unit Delay5/1
  Unit Delay4/1 -> Sum6/1, Sum/2

== system motion/Real Time/X-Y planner /Generate Feedforward Y/Discrete variable delay1 ==
  In1 : Inport  Port=1
  1-alpha : Gain  Gain=1-alpha  Multiplication=Element-wise(K.*u)  SaturateOnIntegerOverflow=on
  Sum1 : Sum  Inputs=++|  SaturateOnIntegerOverflow=on
  Sum2 : Sum  Inputs=+-|  SaturateOnIntegerOverflow=on
  Unit Delay : UnitDelay  X0=0  SampleTime=Ts
  Out1 : Outport  Port=1
  wires:
  Sum2/1 -> 1-alpha/1
  1-alpha/1 -> Sum1/1
  Sum1/1 -> Out1/1
  Unit Delay/1 -> Sum2/2, Sum1/2
  In1/1 -> Unit Delay/1, Sum2/1

== system motion/Real Time/X-Y planner /Generate Feedforward Y/Discrete variable delay2 ==
  In1 : Inport  Port=1
  1-alpha : Gain  Gain=1-alpha  Multiplication=Element-wise(K.*u)  SaturateOnIntegerOverflow=on
  Sum1 : Sum  Inputs=++|  SaturateOnIntegerOverflow=on
  Sum2 : Sum  Inputs=+-|  SaturateOnIntegerOverflow=on
  Unit Delay : UnitDelay  X0=0  SampleTime=Ts
  Out1 : Outport  Port=1
  wires:
  In1/1 -> Sum2/1, Unit Delay/1
  Unit Delay/1 -> Sum1/2, Sum2/2
  Sum1/1 -> Out1/1
  1-alpha/1 -> Sum1/1
  Sum2/1 -> 1-alpha/1

== system motion/Real Time/X-Y planner /Generate Feedforward Y/Discrete variable delay4 ==
  In1 : Inport  Port=1
  1-alpha : Gain  Gain=1-alpha  Multiplication=Element-wise(K.*u)  SaturateOnIntegerOverflow=on
  Sum1 : Sum  Inputs=++|  SaturateOnIntegerOverflow=on
  Sum2 : Sum  Inputs=+-|  SaturateOnIntegerOverflow=on
  Unit Delay : UnitDelay  X0=0  SampleTime=Ts
  Out1 : Outport  Port=1
  wires:
  Sum2/1 -> 1-alpha/1
  1-alpha/1 -> Sum1/1
  Sum1/1 -> Out1/1
  Unit Delay/1 -> Sum2/2, Sum1/2
  In1/1 -> Unit Delay/1, Sum2/1

== system motion/Real Time/X-Y planner /Generate Feedforward Y/acceleration ==
  in : Inport  Port=1
  reset : Inport  Port=2
  Constant : Constant  Value=0
  Constant1 : Constant  Value=0
  Gain4 : Gain  Gain=Ts/2  Multiplication=Element-wise(K.*u)  SaturateOnIntegerOverflow=on
  Sum : Sum  Inputs=|++  SaturateOnIntegerOverflow=on
  Sum1 : Sum  Inputs=|-+  SaturateOnIntegerOverflow=on
  Sum6 : Sum  Inputs=+-  SaturateOnIntegerOverflow=on
  Switch : Switch  Threshold=.5
  Switch1 : Switch  Threshold=.5
  Unit Delay4 : UnitDelay  X0=0  SampleTime=Ts
  Unit Delay5 : UnitDelay  X0=0  SampleTime=Ts
  out : Outport  Port=1
  wires:
  Constant/1 -> Switch/1
  Sum/1 -> Switch/3
  reset/1 -> Switch/2, Switch1/2
  Constant1/1 -> Switch1/1
  Sum1/1 -> Switch1/3
  Gain4/1 -> Sum/1, Sum1/1
  in/1 -> Gain4/1
  Sum6/1 -> out/1
  Unit Delay5/1 -> Sum1/2, Sum6/2
  Switch/1 -> Unit Delay4/1
  Switch1/1 -> Unit Delay5/1
  Unit Delay4/1 -> Sum6/1, Sum/2

== system motion/Real Time/X-Y planner /Generate Feedforward Y/jerk ==
  in : Inport  Port=1
  reset : Inport  Port=2
  Constant : Constant  Value=0
  Constant1 : Constant  Value=0
  Gain4 : Gain  Gain=Ts/2  Multiplication=Element-wise(K.*u)  SaturateOnIntegerOverflow=on
  Sum : Sum  Inputs=|++  SaturateOnIntegerOverflow=on
  Sum1 : Sum  Inputs=|-+  SaturateOnIntegerOverflow=on
  Sum6 : Sum  Inputs=+-  SaturateOnIntegerOverflow=on
  Switch : Switch  Threshold=.5
  Switch1 : Switch  Threshold=.5
  Unit Delay4 : UnitDelay  X0=0  SampleTime=Ts
  Unit Delay5 : UnitDelay  X0=0  SampleTime=Ts
  out : Outport  Port=1
  wires:
  Unit Delay4/1 -> Sum/2, Sum6/1
  Switch1/1 -> Unit Delay5/1
  Switch/1 -> Unit Delay4/1
  Unit Delay5/1 -> Sum6/2, Sum1/2
  Sum6/1 -> out/1
  in/1 -> Gain4/1
  Gain4/1 -> Sum1/1, Sum/1
  Sum1/1 -> Switch1/3
  Constant1/1 -> Switch1/1
  reset/1 -> Switch1/2, Switch/2
  Sum/1 -> Switch/3
  Constant/1 -> Switch/1

== system motion/Real Time/X-Y planner /Generate Feedforward Y/position ==
  in : Inport  Port=1
  reset : Inport  Port=2
  Constant : Constant  Value=0
  Constant1 : Constant  Value=0
  Gain4 : Gain  Gain=Ts/2  Multiplication=Element-wise(K.*u)  SaturateOnIntegerOverflow=on
  Sum : Sum  Inputs=|++  SaturateOnIntegerOverflow=on
  Sum1 : Sum  Inputs=|-+  SaturateOnIntegerOverflow=on
  Sum6 : Sum  Inputs=+-  SaturateOnIntegerOverflow=on
  Switch : Switch  Threshold=.5
  Switch1 : Switch  Threshold=.5
  Unit Delay4 : UnitDelay  X0=0  SampleTime=Ts
  Unit Delay5 : UnitDelay  X0=0  SampleTime=Ts
  out : Outport  Port=1
  wires:
  Constant/1 -> Switch/1
  Sum/1 -> Switch/3
  reset/1 -> Switch/2, Switch1/2
  Constant1/1 -> Switch1/1
  Sum1/1 -> Switch1/3
  Gain4/1 -> Sum/1, Sum1/1
  in/1 -> Gain4/1
  Sum6/1 -> out/1
  Unit Delay5/1 -> Sum1/2, Sum6/2
  Switch/1 -> Unit Delay4/1
  Switch1/1 -> Unit Delay5/1
  Unit Delay4/1 -> Sum6/1, Sum/2

== system motion/Real Time/X-Y planner /Generate Feedforward Y/velocity ==
  in : Inport  Port=1
  reset : Inport  Port=2
  Constant : Constant  Value=0
  Constant1 : Constant  Value=0
  Gain4 : Gain  Gain=Ts/2  Multiplication=Element-wise(K.*u)  SaturateOnIntegerOverflow=on
  Sum : Sum  Inputs=|++  SaturateOnIntegerOverflow=on
  Sum1 : Sum  Inputs=|-+  SaturateOnIntegerOverflow=on
  Sum6 : Sum  Inputs=+-  SaturateOnIntegerOverflow=on
  Switch : Switch  Threshold=.5
  Switch1 : Switch  Threshold=.5
  Unit Delay4 : UnitDelay  X0=0  SampleTime=Ts
  Unit Delay5 : UnitDelay  X0=0  SampleTime=Ts
  out : Outport  Port=1
  wires:
  Unit Delay4/1 -> Sum/2, Sum6/1
  Switch1/1 -> Unit Delay5/1
  Switch/1 -> Unit Delay4/1
  Unit Delay5/1 -> Sum6/2, Sum1/2
  Sum6/1 -> out/1
  in/1 -> Gain4/1
  Gain4/1 -> Sum1/1, Sum/1
  Sum1/1 -> Switch1/3
  Constant1/1 -> Switch1/1
  reset/1 -> Switch1/2, Switch/2
  Sum/1 -> Switch/3
  Constant/1 -> Switch/1
